simulink model "algoritm_3"  (R2017b)
settings: Solver=ode23s  StartTime=0.0  StopTime=200  FixedStep=0.0000001  RelTol=1e-3
values from neighbouring files (symbols this model uses):
  Cwy1 = 0.0074    [Parameters.m]
  Cwy2 = 0.0527    [Parameters.m]
  Cx = 52.92    [Parameters.m]
  Jyy = 0.78    [Parameters.m]
  k1_k = 0.2    [Parameters.m]
  k2_k = 0.1    [Parameters.m]
  k2_m = 2.19    [Parameters.m]
  K_thruster = 2.89    [Parameters.m]
  kc = 57.2958    [Parameters.m]
  L = 1.760    (= 1.76)    [Parameters.m]
  lambda11 = 0.6    [Parameters.m]
  lambda55 = 0.9    [Parameters.m]
  m = 24.7    [Parameters.m]
  Rmin = 0.4    [Parameters.m]
  T_thruster = 0.1    [Parameters.m]
libraries: simulink x6
settings Model: Creator=Eugene  LastModifiedBy=Eugene
settings DebuggingCC: ParameterOverflowMsg=warning
settings HardwareCC: ProdHWDeviceType=AMD->x86-64 (Windows64)

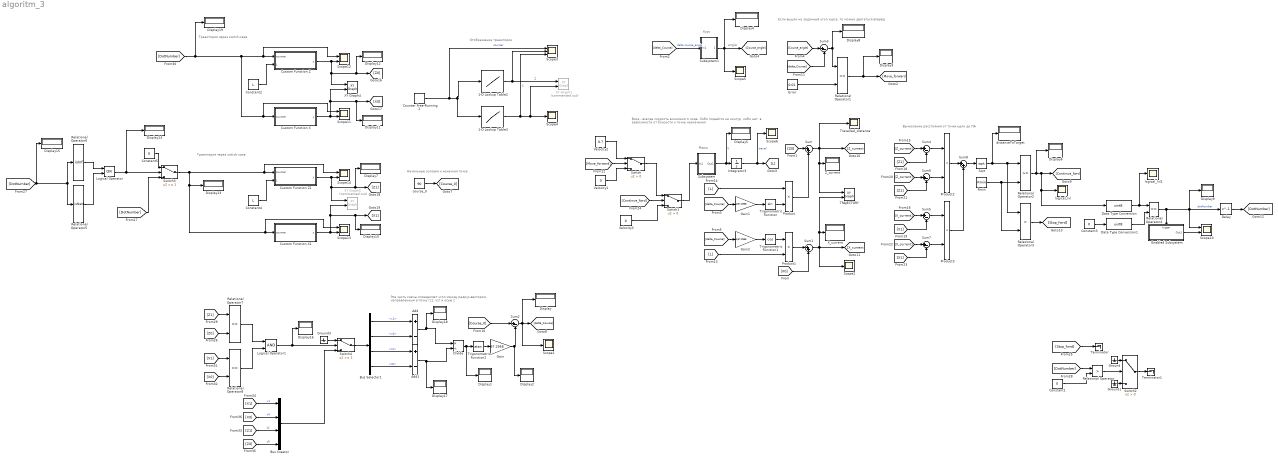
== system algoritm_3 ==
  note: Эта часть схемы определяет угол между радиус-вектором, направленным в точку (z1, x1) и осью z
  note: Вход - всегда скорость экономного хода. Либо подаётся на контур, либо нет, в зависимости от близости к точке назначения
  note: Марш
  note: angle
  note: Курс
  note: Начальные условия и конечная точка
  note: Отображение траектории
  note: Вычисление расстояния от точки-цели до ПА
  note: Если вышли на заданный угол курса, то можно двигаться вперёд
  note: Траектория через switch-case
  note: Траектория через switch-case
  1-D Lookup Table2 : Lookup_n-D  NumberOfTableDimensions=1  BreakpointsForDimension1=[0:7]  BreakpointsForDimension1FirstPoint=0  BreakpointsForDimension1DataTypeStr=uint8  Table=[0,0,L,L,2*L,2*L,3*L, 3*L]  TableDataTypeStr=double  InterpMethod=Flat  ExtrapMethod=Cubic spline  RemoveProtectionInput=on  InternalRulePriority=Speed  OutDataTypeStr=double  RndMeth=Zero  InputSameDT=on
  1-D Lookup Table3 : Lookup_n-D  NumberOfTableDimensions=1  BreakpointsForDimension1=[0:7]  BreakpointsForDimension1DataTypeStr=int16  Table=[0,25,25,0,0,25,25,0]  TableDataTypeStr=double  InterpMethod=Flat  RemoveProtectionInput=on  InternalRulePriority=Speed  OutDataTypeStr=double  RndMeth=Zero  InputSameDT=on
  Add : Sum  Inputs=+-
  Add1 : Sum  Inputs=+-
  Bus Creator : BusCreator  Inputs=4
  Bus Selector1 : BusSelector  OutputSignals=x1,x0,z1,z0
  Constant1 : Constant  Value=0
  Constant2 : Constant  Value=L
  Constant3 : Constant  Value=0
  Constant4 : Constant  Value=L
  Constant5 : Constant  Value=0
  Counter Free-Running2 : simulink/Sources/Counter Free-Running  NumBits=3  tsamp=1
  Custom Function X : MATLAB Function  TreatAsAtomicUnit=on
  Custom Function X1 : MATLAB Function  TreatAsAtomicUnit=on
  Custom Function Z : MATLAB Function  TreatAsAtomicUnit=on
  Custom Function Z1 : MATLAB Function  TreatAsAtomicUnit=on
  Data Type Conversion : DataTypeConversion  OutDataTypeStr=uint8
  Data Type Conversion1 : DataTypeConversion  OutDataTypeStr=uint8
  Delay : Delay  DelayLength=1  SampleTime=4
  Display{,1..19} (20 alike) : Display
  Divide : Product  Inputs=*/
  Enabled Subsystem : Subsystem  TreatAsAtomicUnit=on
  Error : Constant  Value=0.01
  Gain : Gain  Gain=57.2958
  Gain1 : Gain  Gain=1/57.2958
  Gain2 : Gain  Gain=1/57.2958
  Ground : Ground
  Ground1 : Ground
  Ground3 : Ground
  Integrator3 : Integrator
  Logical Operator : Logic  Operator=OR  AllPortsSameDT=off  OutDataTypeStr=boolean
  Logical Operator1 : Logic  AllPortsSameDT=off  OutDataTypeStr=boolean
  Product{,1..3} (4 alike) : Product
  Relational Operator : RelationalOperator  Operator=>  OutDataTypeStr=boolean  RndMeth=Simplest
  Relational Operator1 : RelationalOperator  Operator=<=  OutDataTypeStr=boolean  RndMeth=Simplest
  Relational Operator2 : RelationalOperator  OutDataTypeStr=boolean  RndMeth=Simplest
  Relational Operator3 : RelationalOperator  Operator=<  OutDataTypeStr=boolean  RndMeth=Simplest
  Relational Operator4 : RelationalOperator  Operator===  OutDataTypeStr=boolean  RndMeth=Simplest
  Relational Operator5 : RelationalOperator  Operator=isNaN  OutDataTypeStr=boolean  RndMeth=Simplest
  Relational Operator6 : RelationalOperator  Operator=isInf  OutDataTypeStr=boolean  RndMeth=Simplest
  Relational Operator7 : RelationalOperator  Operator===  OutDataTypeStr=boolean  RndMeth=Simplest
  Relational Operator8 : RelationalOperator  Operator===  OutDataTypeStr=boolean  RndMeth=Simplest
  Rmin : Constant  Value=Rmin
  Scope{1..2,4..6} (5 alike) : Scope
  Scope{10..14} (5 alike) : Scope  NumInputPorts=2
  Scope3 : Scope  NumInputPorts=3
  Sqrt : Sqrt  SaturateOnIntegerOverflow=on
  Subsystem : Subsystem
  Subsystem1 : Subsystem
  Sum : Sum  Inputs=|++
  Sum1 : Sum  Inputs=|++
  Sum{2..7} (6 alike) : Sum  Inputs=|+-
  Sum8 : Sum  Inputs=|++
  Switch : Switch  Criteria=u2 > Threshold
  Switch1 : Switch  Criteria=u2 > Threshold
  Switch2 : Switch  Criteria=u2 > Threshold
  Switch3 : Switch  Threshold=1
  Switch4 : Switch  Threshold=1
  TRAJECTORY : simulink/Sinks/XY Graph  xmin=-5  xmax=30  ymin=-5  ymax=30  st=-1
  Terminator : Terminator
  Terminator1 : Terminator
  Travelled_distance : Scope
  Trigonometric Function : Trigonometry
  Trigonometric Function1 : Trigonometry  Operator=cos
  Trigonometric Function2 : Trigonometry  Operator=atan  OutputSignalType=real
  Velocity1 : Constant  Value=0
  Velocity2 : Constant  Value=0.7
  Velocity3 : Constant  Value=0
  XY Graph1 : simulink/Sinks/XY Graph  Commented=on  xmin=-10  xmax=20  ymin=-10  ymax=30  st=-1
  XY Graph4 : simulink/Sinks/XY Graph  xmin=-10  xmax=20  ymin=-10  ymax=30  st=-1
  XY Graph5 : simulink/Sinks/XY Graph  Commented=on  xmin=-10  xmax=20  ymin=-10  ymax=30  st=-1
  X_current : Display
  Z_current : Display
  "course_0 " : Constant  Value=90
  distanceToTarget : Display
  logical_lvl : Scope
  logical_lvl1 : Scope
  wires:
  1-D Lookup Table3/1 -> Scope4/1, XY Graph1/2, Scope3/3  "X"
  1-D Lookup Table2/1 -> XY Graph1/1, Scope3/2  "Z"
  Counter Free-Running2/1 -> Scope3/1, 1-D Lookup Table2/1, 1-D Lookup Table3/1  "counter"
  Subsystem/1(Out1) -> Display5/1, Integrator3/1  "V"
  [delta_Course] -> Subsystem1/1(In1)  "delta course_angle"
  Subsystem1/1(Out1) -> Display4/1, Scope5/1, [Course_angle]
  Product/1 -> Sum/2
  Sum/1 -> TRAJECTORY/1, Z_current/1, [Z_current], Travelled_distance/1
  Product1/1 -> Sum1/1
  Sum1/1 -> [X_current], Scope2/1, TRAJECTORY/2, X_current/1
  Trigonometric Function/1 -> Product/2
  [Z0] -> Sum/1
  [delta_Course] -> Gain1/1
  [delta_Course] -> Gain2/1
  Trigonometric Function1/1 -> Product1/1
  [X0] -> Sum1/2
  Integrator3/1 -> Scope6/1, [L]  "travel"
  Divide/1 -> Display1/1, Trigonometric Function2/1
  "course_0 "/1 -> [Course_0]
  [Course_0] -> Sum2/1
  Trigonometric Function2/1 -> Gain/1
  Sum2/1 -> Scope1/1, Display/1, [delta_Course]
  Gain/1 -> Display2/1, Sum2/2
  [Course_angle] -> Sum3/1
  [delta_Course] -> Sum3/2
  Velocity2/1 -> Switch/1
  Velocity1/1 -> Switch/3
  Sum3/1 -> Display8/1, Relational Operator1/1
  Error/1 -> Relational Operator1/2
  Relational Operator1/1 -> [Move_forward], Display3/1
  [Move_forward] -> Switch/2
  [L] -> Product1/2
  [L] -> Product/1
  Gain1/1 -> Trigonometric Function/1
  Gain2/1 -> Trigonometric Function1/1
  [Z_current] -> Sum4/1
  [Z1] -> Sum4/2
  [X_current] -> Sum5/1
  [X1] -> Sum5/2
  [Z1] -> Sum6/2
  [Z_current] -> Sum6/1
  Sum4/1 -> Product2/1
  Sum6/1 -> Product2/2
  Sum5/1 -> Product3/1
  Sum7/1 -> Product3/2
  [X1] -> Sum7/2
  [X_current] -> Sum7/1
  Product2/1 -> Sum8/1
  Product3/1 -> Sum8/2
  Sum8/1 -> Sqrt/1
  Sqrt/1 -> Relational Operator2/1, Relational Operator3/1, distanceToTarget/1
  Rmin/1 -> Relational Operator2/2, Relational Operator3/2
  Relational Operator2/1 -> Data Type Conversion/1, logical_lvl/1, [Continue_fwrd], Display6/1
  Relational Operator3/1 -> [Stop_fwrd]
  [Continue_fwrd] -> Switch1/2
  Switch/1 -> Switch1/1
  Switch1/1 -> Subsystem/1(In1)
  Velocity3/1 -> Switch1/3
  [Stop_fwrd] -> Terminator/1
  Data Type Conversion/1 -> logical_lvl1/1, Relational Operator4/1
  Constant3/1 -> Data Type Conversion1/1
  Data Type Conversion1/1 -> Relational Operator4/2
  Enabled Subsystem/1(Out1) -> Scope10/2
  [DotNumber] -> Relational Operator/1
  Constant1/1 -> Relational Operator/2
  Relational Operator/1 -> Switch2/2
  Custom Function X1/1(y) -> Display10/1, [X1], XY Graph5/2, Scope13/2
  Custom Function Z1/1(y) -> Scope14/2, Display7/1, [Z1], XY Graph5/1
  Custom Function Z/1(y) -> Display12/1, [Z0], XY Graph4/1, Scope12/2
  Constant2/1 -> Custom Function Z/2(L)
  Constant4/1 -> Custom Function Z1/2(L)
  Custom Function X/1(y) -> Scope11/2, Display11/1, [X0], XY Graph4/2
  Switch2/1 -> Terminator1/1
  Ground/1 -> Switch2/1
  Ground1/1 -> Switch2/3
  Relational Operator4/1 -> Delay/1, Scope10/1, Display9/1, Enabled Subsystem/Trigger  "dotNumber"
  [DotNumber] -> Display19/1, Custom Function X/1(counter), Scope11/1, Scope12/1, Custom Function Z/1(counter)
  [DotNumber] -> Display15/1, Relational Operator6/1, Relational Operator5/1
  Switch3/1 -> Display13/1, Scope13/1, Custom Function X1/1(counter), Scope14/1, Custom Function Z1/1(counter)
  Constant5/1 -> Switch3/1
  [DotNumber] -> Switch3/3
  Relational Operator6/1 -> Logical Operator/1
  Relational Operator5/1 -> Logical Operator/2
  Logical Operator/1 -> Switch3/2, Display14/1
  Add1/1 -> Display17/1, Divide/2
  Add/1 -> Display18/1, Divide/1
  [Z1] -> Relational Operator7/1
  [Z0] -> Relational Operator7/2
  [X1] -> Relational Operator8/1
  [X0] -> Relational Operator8/2
  Relational Operator7/1 -> Logical Operator1/1
  Relational Operator8/1 -> Logical Operator1/2
  Logical Operator1/1 -> Display16/1, Switch4/2
  Bus Creator/1 -> Switch4/3
  Switch4/1 -> Bus Selector1/1
  [Z0] -> Bus Creator/4  "z0"
  [Z1] -> Bus Creator/3  "z1"
  [X1] -> Bus Creator/1  "x1"
  [X0] -> Bus Creator/2  "x0"
  Ground3/1 -> Switch4/1
  Delay/1 -> [DotNumber]
  Bus Selector1/1 -> Add/1  "<x1>"
  Bus Selector1/2 -> Add/2  "<x0>"
  Bus Selector1/3 -> Add1/1  "<z1>"
  Bus Selector1/4 -> Add1/2  "<z0>"

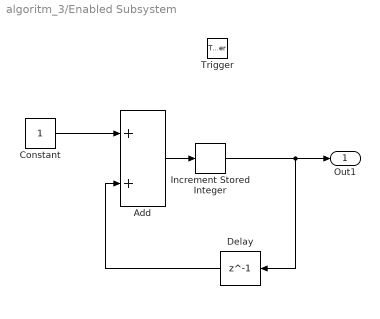
== system algoritm_3/Enabled Subsystem ==
  Trigger : TriggerPort  TriggerType=falling  VariantControl=Variant  PortDimensions=1
  Add : Sum
  Constant : Constant
  Delay : Delay  DelayLength=1  InitialCondition=0
  Increment Stored Integer : simulink/Additional Math & Discrete/Additional Math: Increment - Decrement/Increment Stored Integer
      settings: SourceProductName=Simulink
  Out1 : Outport
  wires:
  Constant/1 -> Add/1
  Delay/1 -> Add/2
  Add/1 -> Increment Stored Integer/1
  Increment Stored Integer/1 -> Delay/1, Out1/1

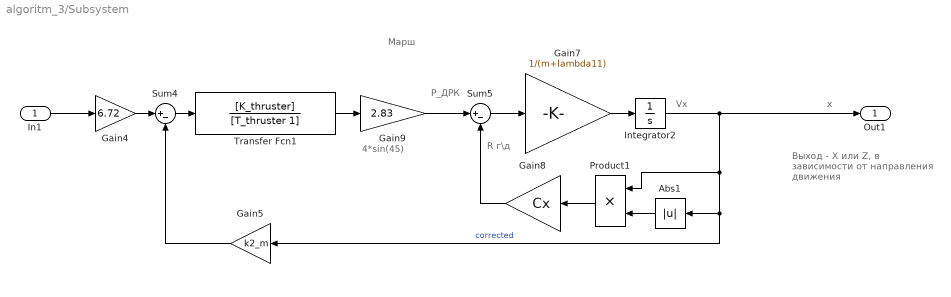
== system algoritm_3/Subsystem ==
  note: Выход - X или Z, в зависимости от направления движения
  note: 4*sin(45)
  note: R г\д
  note: x
  note: Vx
  note: P_ДРК
  note: Марш
  In1 : Inport
  Abs1 : Abs
  Gain4 : Gain  Gain=6.72
  Gain5 : Gain  Gain=k2_m
  Gain7 : Gain  Gain=1/(m+lambda11)
  Gain8 : Gain  Gain=Cx
  Gain9 : Gain  Gain=2.83
  Integrator2 : Integrator
  Product1 : Product
  Sum4 : Sum  Inputs=|+-
  Sum5 : Sum  Inputs=|+-
  Transfer Fcn1 : TransferFcn  Numerator=[K_thruster]  Denominator=[T_thruster 1]
  Out1 : Outport
  wires:
  In1/1 -> Gain4/1
  Product1/1 -> Gain8/1
  Gain7/1 -> Integrator2/1
  Gain8/1 -> Sum5/2
  Integrator2/1 -> Out1/1, Gain5/1, Abs1/1, Product1/1  "corrected"
  Transfer Fcn1/1 -> Gain9/1
  Gain4/1 -> Sum4/1
  Sum4/1 -> Transfer Fcn1/1
  Sum5/1 -> Gain7/1
  Gain9/1 -> Sum5/1
  Gain5/1 -> Sum4/2
  Abs1/1 -> Product1/2

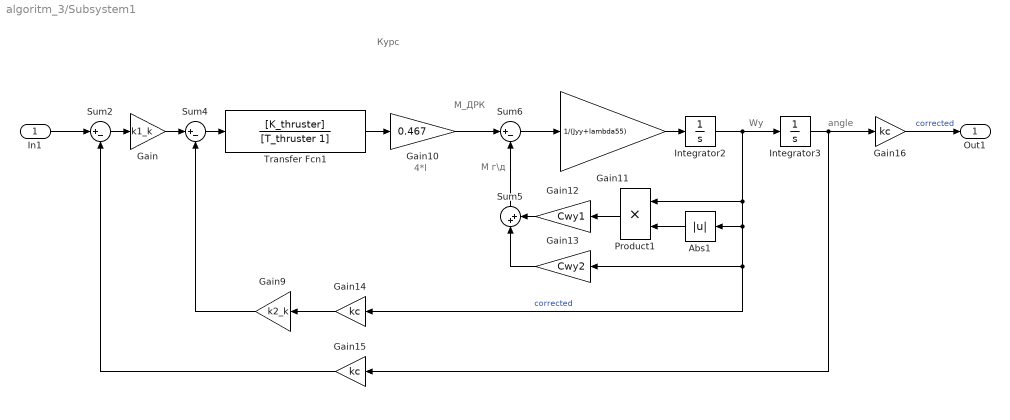
== system algoritm_3/Subsystem1 ==
  note: Курс
  note: Wy
  note: M_ДРК
  note: 4*l
  note: angle
  note: M г\д
  In1 : Inport
  Abs1 : Abs
  Gain : Gain  Gain=k1_k
  Gain10 : Gain  Gain=0.467
  Gain11 : Gain  Gain=1/(Jyy+lambda55)
  Gain12 : Gain  Gain=Cwy1
  Gain13 : Gain  Gain=Cwy2
  Gain14 : Gain  Gain=kc
  Gain15 : Gain  Gain=kc
  Gain16 : Gain  Gain=kc
  Gain9 : Gain  Gain=k2_k
  Integrator2 : Integrator
  Integrator3 : Integrator
  Product1 : Product
  Sum2 : Sum  Inputs=|+-
  Sum4 : Sum  Inputs=|+-
  Sum5 : Sum  Inputs=|++
  Sum6 : Sum  Inputs=|+-
  Transfer Fcn1 : TransferFcn  Numerator=[K_thruster]  Denominator=[T_thruster 1]
  Out1 : Outport
  wires:
  Gain12/1 -> Sum5/2
  Gain10/1 -> Sum6/1
  Product1/1 -> Gain12/1
  Gain11/1 -> Integrator2/1
  Gain9/1 -> Sum4/2
  Gain/1 -> Sum4/1
  Transfer Fcn1/1 -> Gain10/1
  Sum6/1 -> Gain11/1
  Gain14/1 -> Gain9/1
  Gain15/1 -> Sum2/2
  Gain13/1 -> Sum5/1
  Abs1/1 -> Product1/2
  Sum5/1 -> Sum6/2
  Integrator2/1 -> Gain14/1, Gain13/1, Abs1/1, Product1/1, Integrator3/1  "corrected"
  Sum2/1 -> Gain/1
  Integrator3/1 -> Gain16/1, Gain15/1
  Sum4/1 -> Transfer Fcn1/1
  In1/1 -> Sum2/1
  Gain16/1 -> Out1/1  "corrected"

== matlab function algoritm_3/Custom Function X ==
  data: counter input; y output
function y = fcn(counter)

%L = 1.76;

switch counter
    case 1
      y = 25;
    case 2
      y = 25;
    case 3
      y = 0;
    case 4
      y = 0;
    case 5
      y = 25;
    case 6
      y = 25;
    case 7
      y = 0;
    case 8
      y = 0;
    case 9
      y = 25;      
   otherwise
      y = 0;
end

== matlab function algoritm_3/Custom Function Z ==
  data: counter input; y output; L input
function y = fcn(counter, L)

%L = 1.76;

switch counter
    case 1
      y = 0;
    case 2
      y = L;
    case 3
      y = L;
    case 4
      y = 2*L;
    case 5
      y = 2*L;
    case 6
      y = 3*L;
    case 7
      y = 3*L;
    case 8
      y = 4*L;
    case 9
      y = 4*L;      
   otherwise
      y = 0;
end

== matlab function algoritm_3/Custom Function X1 ==
  data: counter input; y output
function y = fcn(counter)

%L = 1.76;

switch counter
    case 1
      y = 25;
    case 2
      y = 0;
    case 3
      y = 0;
    case 4
      y = 25;
    case 5
      y = 25;
    case 6
      y = 0;
    case 7
      y = 0;
    case 8
      y = 25;    
    case 9
      y = 25;
   otherwise
      y = 25;
end

== matlab function algoritm_3/Custom Function Z1 ==
  data: counter input; y output; L input
function y = fcn( counter, L)

%L = 1.76;

switch counter
    case 1
      y = L;
    case 2
      y = L;
    case 3
      y = 2*L;
    case 4
      y = 2*L;
    case 5
      y = 3*L;
    case 6
      y = 3*L;
    case 7
      y = 4*L;
    case 8
      y = 4*L;      
    case 9
      y = 5*L;      
   otherwise
      y = 0;
end
